simulink model "gm_ZynqBF_2tx_fpga"  (R2018b)
settings: Solver=FixedStepDiscrete  StartTime=0.0  StopTime=10.0  FixedStep=(1/420e3)/128  RelTol=1e-3
undefined symbols (not defined in the file or in its folder): a, b, c
libraries: hdlsllib x873, simulink x349
(part 21 of 40)

== system gm_ZynqBF_2tx_fpga/channel_estimator/peakdetect_ch1/correlator1/rx_ram_q_instance60 ==
  i : Inport  OutDataTypeStr=fixdt(0, 6, 0)  PortDimensions=1  SampleTime=1.86011904761905e-08
  wdata : Inport  Port=2  OutDataTypeStr=fixdt(1, 16, 15)  PortDimensions=1  SampleTime=1.86011904761905e-08
  waddr : Inport  Port=3  OutDataTypeStr=fixdt(0, 9, 0)  PortDimensions=1  SampleTime=1.86011904761905e-08
  we : Inport  Port=4  OutDataTypeStr=fixdt(0, 64, 0)  PortDimensions=1  SampleTime=1.86011904761905e-08
  raddr : Inport  Port=5  OutDataTypeStr=fixdt(0, 10, 0)  PortDimensions=1  SampleTime=1.86011904761905e-08
  shift : Inport  Port=6  OutDataTypeStr=fixdt(0, 6, 0)  PortDimensions=1  SampleTime=1.86011904761905e-08
  Constant : Constant  OutDataTypeStr=fixdt(0, 1, 0)  SampleTime=-1
  Constant1 : Constant  OutDataTypeStr=fixdt(0, 1, 0)  SampleTime=-1
  Relational Operator : RelationalOperator  Operator=<  OutDataTypeStr=boolean  SampleTime=1.86011904761905e-08  RndMeth=Nearest
  Simple Dual Port RAM : hdlsllib/HDL RAMs/Simple Dual Port RAM  ram_size=9
      settings: SourceProductName=HDL Coder  SourceProductBaseCode=HD
  Sum : Sum  AccumDataTypeStr=fixdt(0, 11, 0)  OutDataTypeStr=fixdt(0, 9, 0)  SampleTime=1.86011904761905e-08
  Sum1 : Sum  AccumDataTypeStr=fixdt(0, 7, 0)  OutDataTypeStr=fixdt(0, 9, 0)  SampleTime=1.86011904761905e-08
  Switch : Switch  Criteria=u2 ~= 0  Threshold=double(0)  OutDataTypeStr=fixdt(0, 9, 0)  SampleTime=1.86011904761905e-08
  get_bit : Subsystem
  dout : Outport
  probe : Outport  Port=2
  wires:
  shift/1 -> Relational Operator/2
  raddr/1 -> Switch/3, Sum/2
  we/1 -> get_bit/1(u)
  waddr/1 -> Simple Dual Port RAM/2
  wdata/1 -> Simple Dual Port RAM/1
  i/1 -> Sum1/1, Relational Operator/1
  Constant/1 -> Sum/1
  Constant1/1 -> Sum1/2
  Relational Operator/1 -> Switch/2
  Simple Dual Port RAM/1 -> dout/1
  Sum/1 -> Switch/1
  Sum1/1 -> get_bit/2(ind)
  Switch/1 -> Simple Dual Port RAM/4, probe/1
  get_bit/1(y) -> Simple Dual Port RAM/3

== system gm_ZynqBF_2tx_fpga/channel_estimator/peakdetect_ch1/correlator1/rx_ram_q_instance61 ==
  i : Inport  OutDataTypeStr=fixdt(0, 6, 0)  PortDimensions=1  SampleTime=1.86011904761905e-08
  wdata : Inport  Port=2  OutDataTypeStr=fixdt(1, 16, 15)  PortDimensions=1  SampleTime=1.86011904761905e-08
  waddr : Inport  Port=3  OutDataTypeStr=fixdt(0, 9, 0)  PortDimensions=1  SampleTime=1.86011904761905e-08
  we : Inport  Port=4  OutDataTypeStr=fixdt(0, 64, 0)  PortDimensions=1  SampleTime=1.86011904761905e-08
  raddr : Inport  Port=5  OutDataTypeStr=fixdt(0, 10, 0)  PortDimensions=1  SampleTime=1.86011904761905e-08
  shift : Inport  Port=6  OutDataTypeStr=fixdt(0, 6, 0)  PortDimensions=1  SampleTime=1.86011904761905e-08
  Constant : Constant  OutDataTypeStr=fixdt(0, 1, 0)  SampleTime=-1
  Constant1 : Constant  OutDataTypeStr=fixdt(0, 1, 0)  SampleTime=-1
  Relational Operator : RelationalOperator  Operator=<  OutDataTypeStr=boolean  SampleTime=1.86011904761905e-08  RndMeth=Nearest
  Simple Dual Port RAM : hdlsllib/HDL RAMs/Simple Dual Port RAM  ram_size=9
      settings: SourceProductName=HDL Coder  SourceProductBaseCode=HD
  Sum : Sum  AccumDataTypeStr=fixdt(0, 11, 0)  OutDataTypeStr=fixdt(0, 9, 0)  SampleTime=1.86011904761905e-08
  Sum1 : Sum  AccumDataTypeStr=fixdt(0, 7, 0)  OutDataTypeStr=fixdt(0, 9, 0)  SampleTime=1.86011904761905e-08
  Switch : Switch  Criteria=u2 ~= 0  Threshold=double(0)  OutDataTypeStr=fixdt(0, 9, 0)  SampleTime=1.86011904761905e-08
  get_bit : Subsystem
  dout : Outport
  probe : Outport  Port=2
  wires:
  shift/1 -> Relational Operator/2
  raddr/1 -> Switch/3, Sum/2
  we/1 -> get_bit/1(u)
  waddr/1 -> Simple Dual Port RAM/2
  wdata/1 -> Simple Dual Port RAM/1
  i/1 -> Sum1/1, Relational Operator/1
  Constant/1 -> Sum/1
  Constant1/1 -> Sum1/2
  Relational Operator/1 -> Switch/2
  Simple Dual Port RAM/1 -> dout/1
  Sum/1 -> Switch/1
  Sum1/1 -> get_bit/2(ind)
  Switch/1 -> Simple Dual Port RAM/4, probe/1
  get_bit/1(y) -> Simple Dual Port RAM/3

== system gm_ZynqBF_2tx_fpga/channel_estimator/peakdetect_ch1/correlator1/rx_ram_q_instance62 ==
  i : Inport  OutDataTypeStr=fixdt(0, 6, 0)  PortDimensions=1  SampleTime=1.86011904761905e-08
  wdata : Inport  Port=2  OutDataTypeStr=fixdt(1, 16, 15)  PortDimensions=1  SampleTime=1.86011904761905e-08
  waddr : Inport  Port=3  OutDataTypeStr=fixdt(0, 9, 0)  PortDimensions=1  SampleTime=1.86011904761905e-08
  we : Inport  Port=4  OutDataTypeStr=fixdt(0, 64, 0)  PortDimensions=1  SampleTime=1.86011904761905e-08
  raddr : Inport  Port=5  OutDataTypeStr=fixdt(0, 10, 0)  PortDimensions=1  SampleTime=1.86011904761905e-08
  shift : Inport  Port=6  OutDataTypeStr=fixdt(0, 6, 0)  PortDimensions=1  SampleTime=1.86011904761905e-08
  Constant : Constant  OutDataTypeStr=fixdt(0, 1, 0)  SampleTime=-1
  Constant1 : Constant  OutDataTypeStr=fixdt(0, 1, 0)  SampleTime=-1
  Relational Operator : RelationalOperator  Operator=<  OutDataTypeStr=boolean  SampleTime=1.86011904761905e-08  RndMeth=Nearest
  Simple Dual Port RAM : hdlsllib/HDL RAMs/Simple Dual Port RAM  ram_size=9
      settings: SourceProductName=HDL Coder  SourceProductBaseCode=HD
  Sum : Sum  AccumDataTypeStr=fixdt(0, 11, 0)  OutDataTypeStr=fixdt(0, 9, 0)  SampleTime=1.86011904761905e-08
  Sum1 : Sum  AccumDataTypeStr=fixdt(0, 7, 0)  OutDataTypeStr=fixdt(0, 9, 0)  SampleTime=1.86011904761905e-08
  Switch : Switch  Criteria=u2 ~= 0  Threshold=double(0)  OutDataTypeStr=fixdt(0, 9, 0)  SampleTime=1.86011904761905e-08
  get_bit : Subsystem
  dout : Outport
  probe : Outport  Port=2
  wires:
  shift/1 -> Relational Operator/2
  raddr/1 -> Switch/3, Sum/2
  we/1 -> get_bit/1(u)
  waddr/1 -> Simple Dual Port RAM/2
  wdata/1 -> Simple Dual Port RAM/1
  i/1 -> Sum1/1, Relational Operator/1
  Constant/1 -> Sum/1
  Constant1/1 -> Sum1/2
  Relational Operator/1 -> Switch/2
  Simple Dual Port RAM/1 -> dout/1
  Sum/1 -> Switch/1
  Sum1/1 -> get_bit/2(ind)
  Switch/1 -> Simple Dual Port RAM/4, probe/1
  get_bit/1(y) -> Simple Dual Port RAM/3

== system gm_ZynqBF_2tx_fpga/channel_estimator/peakdetect_ch1/correlator1/rx_ram_q_instance63 ==
  i : Inport  OutDataTypeStr=fixdt(0, 6, 0)  PortDimensions=1  SampleTime=1.86011904761905e-08
  wdata : Inport  Port=2  OutDataTypeStr=fixdt(1, 16, 15)  PortDimensions=1  SampleTime=1.86011904761905e-08
  waddr : Inport  Port=3  OutDataTypeStr=fixdt(0, 9, 0)  PortDimensions=1  SampleTime=1.86011904761905e-08
  we : Inport  Port=4  OutDataTypeStr=fixdt(0, 64, 0)  PortDimensions=1  SampleTime=1.86011904761905e-08
  raddr : Inport  Port=5  OutDataTypeStr=fixdt(0, 10, 0)  PortDimensions=1  SampleTime=1.86011904761905e-08
  shift : Inport  Port=6  OutDataTypeStr=fixdt(0, 6, 0)  PortDimensions=1  SampleTime=1.86011904761905e-08
  Constant : Constant  OutDataTypeStr=fixdt(0, 1, 0)  SampleTime=-1
  Constant1 : Constant  OutDataTypeStr=fixdt(0, 1, 0)  SampleTime=-1
  Relational Operator : RelationalOperator  Operator=<  OutDataTypeStr=boolean  SampleTime=1.86011904761905e-08  RndMeth=Nearest
  Simple Dual Port RAM : hdlsllib/HDL RAMs/Simple Dual Port RAM  ram_size=9
      settings: SourceProductName=HDL Coder  SourceProductBaseCode=HD
  Sum : Sum  AccumDataTypeStr=fixdt(0, 11, 0)  OutDataTypeStr=fixdt(0, 9, 0)  SampleTime=1.86011904761905e-08
  Sum1 : Sum  AccumDataTypeStr=fixdt(0, 7, 0)  OutDataTypeStr=fixdt(0, 9, 0)  SampleTime=1.86011904761905e-08
  Switch : Switch  Criteria=u2 ~= 0  Threshold=double(0)  OutDataTypeStr=fixdt(0, 9, 0)  SampleTime=1.86011904761905e-08
  get_bit : Subsystem
  dout : Outport
  probe : Outport  Port=2
  wires:
  shift/1 -> Relational Operator/2
  raddr/1 -> Switch/3, Sum/2
  we/1 -> get_bit/1(u)
  waddr/1 -> Simple Dual Port RAM/2
  wdata/1 -> Simple Dual Port RAM/1
  i/1 -> Sum1/1, Relational Operator/1
  Constant/1 -> Sum/1
  Constant1/1 -> Sum1/2
  Relational Operator/1 -> Switch/2
  Simple Dual Port RAM/1 -> dout/1
  Sum/1 -> Switch/1
  Sum1/1 -> get_bit/2(ind)
  Switch/1 -> Simple Dual Port RAM/4, probe/1
  get_bit/1(y) -> Simple Dual Port RAM/3

== system gm_ZynqBF_2tx_fpga/channel_estimator/peakdetect_ch1/correlator1/rx_ram_q_instance64 ==
  i : Inport  OutDataTypeStr=fixdt(0, 6, 0)  PortDimensions=1  SampleTime=1.86011904761905e-08
  wdata : Inport  Port=2  OutDataTypeStr=fixdt(1, 16, 15)  PortDimensions=1  SampleTime=1.86011904761905e-08
  waddr : Inport  Port=3  OutDataTypeStr=fixdt(0, 9, 0)  PortDimensions=1  SampleTime=1.86011904761905e-08
  we : Inport  Port=4  OutDataTypeStr=fixdt(0, 64, 0)  PortDimensions=1  SampleTime=1.86011904761905e-08
  raddr : Inport  Port=5  OutDataTypeStr=fixdt(0, 10, 0)  PortDimensions=1  SampleTime=1.86011904761905e-08
  shift : Inport  Port=6  OutDataTypeStr=fixdt(0, 6, 0)  PortDimensions=1  SampleTime=1.86011904761905e-08
  Constant : Constant  OutDataTypeStr=fixdt(0, 1, 0)  SampleTime=-1
  Constant1 : Constant  OutDataTypeStr=fixdt(0, 1, 0)  SampleTime=-1
  Relational Operator : RelationalOperator  Operator=<  OutDataTypeStr=boolean  SampleTime=1.86011904761905e-08  RndMeth=Nearest
  Simple Dual Port RAM : hdlsllib/HDL RAMs/Simple Dual Port RAM  ram_size=9
      settings: SourceProductName=HDL Coder  SourceProductBaseCode=HD
  Sum : Sum  AccumDataTypeStr=fixdt(0, 11, 0)  OutDataTypeStr=fixdt(0, 9, 0)  SampleTime=1.86011904761905e-08
  Sum1 : Sum  AccumDataTypeStr=fixdt(0, 7, 0)  OutDataTypeStr=fixdt(0, 9, 0)  SampleTime=1.86011904761905e-08
  Switch : Switch  Criteria=u2 ~= 0  Threshold=double(0)  OutDataTypeStr=fixdt(0, 9, 0)  SampleTime=1.86011904761905e-08
  get_bit : Subsystem
  dout : Outport
  probe : Outport  Port=2
  wires:
  shift/1 -> Relational Operator/2
  raddr/1 -> Switch/3, Sum/2
  we/1 -> get_bit/1(u)
  waddr/1 -> Simple Dual Port RAM/2
  wdata/1 -> Simple Dual Port RAM/1
  i/1 -> Sum1/1, Relational Operator/1
  Constant/1 -> Sum/1
  Constant1/1 -> Sum1/2
  Relational Operator/1 -> Switch/2
  Simple Dual Port RAM/1 -> dout/1
  Sum/1 -> Switch/1
  Sum1/1 -> get_bit/2(ind)
  Switch/1 -> Simple Dual Port RAM/4, probe/1
  get_bit/1(y) -> Simple Dual Port RAM/3

== system gm_ZynqBF_2tx_fpga/channel_estimator/peakdetect_ch1/correlator1/rx_ram_q_instance7 ==
  i : Inport  OutDataTypeStr=fixdt(0, 6, 0)  PortDimensions=1  SampleTime=1.86011904761905e-08
  wdata : Inport  Port=2  OutDataTypeStr=fixdt(1, 16, 15)  PortDimensions=1  SampleTime=1.86011904761905e-08
  waddr : Inport  Port=3  OutDataTypeStr=fixdt(0, 9, 0)  PortDimensions=1  SampleTime=1.86011904761905e-08
  we : Inport  Port=4  OutDataTypeStr=fixdt(0, 64, 0)  PortDimensions=1  SampleTime=1.86011904761905e-08
  raddr : Inport  Port=5  OutDataTypeStr=fixdt(0, 10, 0)  PortDimensions=1  SampleTime=1.86011904761905e-08
  shift : Inport  Port=6  OutDataTypeStr=fixdt(0, 6, 0)  PortDimensions=1  SampleTime=1.86011904761905e-08
  Constant : Constant  OutDataTypeStr=fixdt(0, 1, 0)  SampleTime=-1
  Constant1 : Constant  OutDataTypeStr=fixdt(0, 1, 0)  SampleTime=-1
  Relational Operator : RelationalOperator  Operator=<  OutDataTypeStr=boolean  SampleTime=1.86011904761905e-08  RndMeth=Nearest
  Simple Dual Port RAM : hdlsllib/HDL RAMs/Simple Dual Port RAM  ram_size=9
      settings: SourceProductName=HDL Coder  SourceProductBaseCode=HD
  Sum : Sum  AccumDataTypeStr=fixdt(0, 11, 0)  OutDataTypeStr=fixdt(0, 9, 0)  SampleTime=1.86011904761905e-08
  Sum1 : Sum  AccumDataTypeStr=fixdt(0, 7, 0)  OutDataTypeStr=fixdt(0, 9, 0)  SampleTime=1.86011904761905e-08
  Switch : Switch  Criteria=u2 ~= 0  Threshold=double(0)  OutDataTypeStr=fixdt(0, 9, 0)  SampleTime=1.86011904761905e-08
  get_bit : Subsystem
  dout : Outport
  probe : Outport  Port=2
  wires:
  shift/1 -> Relational Operator/2
  raddr/1 -> Switch/3, Sum/2
  we/1 -> get_bit/1(u)
  waddr/1 -> Simple Dual Port RAM/2
  wdata/1 -> Simple Dual Port RAM/1
  i/1 -> Sum1/1, Relational Operator/1
  Constant/1 -> Sum/1
  Constant1/1 -> Sum1/2
  Relational Operator/1 -> Switch/2
  Simple Dual Port RAM/1 -> dout/1
  Sum/1 -> Switch/1
  Sum1/1 -> get_bit/2(ind)
  Switch/1 -> Simple Dual Port RAM/4, probe/1
  get_bit/1(y) -> Simple Dual Port RAM/3

== system gm_ZynqBF_2tx_fpga/channel_estimator/peakdetect_ch1/correlator1/rx_ram_q_instance8 ==
  i : Inport  OutDataTypeStr=fixdt(0, 6, 0)  PortDimensions=1  SampleTime=1.86011904761905e-08
  wdata : Inport  Port=2  OutDataTypeStr=fixdt(1, 16, 15)  PortDimensions=1  SampleTime=1.86011904761905e-08
  waddr : Inport  Port=3  OutDataTypeStr=fixdt(0, 9, 0)  PortDimensions=1  SampleTime=1.86011904761905e-08
  we : Inport  Port=4  OutDataTypeStr=fixdt(0, 64, 0)  PortDimensions=1  SampleTime=1.86011904761905e-08
  raddr : Inport  Port=5  OutDataTypeStr=fixdt(0, 10, 0)  PortDimensions=1  SampleTime=1.86011904761905e-08
  shift : Inport  Port=6  OutDataTypeStr=fixdt(0, 6, 0)  PortDimensions=1  SampleTime=1.86011904761905e-08
  Constant : Constant  OutDataTypeStr=fixdt(0, 1, 0)  SampleTime=-1
  Constant1 : Constant  OutDataTypeStr=fixdt(0, 1, 0)  SampleTime=-1
  Relational Operator : RelationalOperator  Operator=<  OutDataTypeStr=boolean  SampleTime=1.86011904761905e-08  RndMeth=Nearest
  Simple Dual Port RAM : hdlsllib/HDL RAMs/Simple Dual Port RAM  ram_size=9
      settings: SourceProductName=HDL Coder  SourceProductBaseCode=HD
  Sum : Sum  AccumDataTypeStr=fixdt(0, 11, 0)  OutDataTypeStr=fixdt(0, 9, 0)  SampleTime=1.86011904761905e-08
  Sum1 : Sum  AccumDataTypeStr=fixdt(0, 7, 0)  OutDataTypeStr=fixdt(0, 9, 0)  SampleTime=1.86011904761905e-08
  Switch : Switch  Criteria=u2 ~= 0  Threshold=double(0)  OutDataTypeStr=fixdt(0, 9, 0)  SampleTime=1.86011904761905e-08
  get_bit : Subsystem
  dout : Outport
  probe : Outport  Port=2
  wires:
  shift/1 -> Relational Operator/2
  raddr/1 -> Switch/3, Sum/2
  we/1 -> get_bit/1(u)
  waddr/1 -> Simple Dual Port RAM/2
  wdata/1 -> Simple Dual Port RAM/1
  i/1 -> Sum1/1, Relational Operator/1
  Constant/1 -> Sum/1
  Constant1/1 -> Sum1/2
  Relational Operator/1 -> Switch/2
  Simple Dual Port RAM/1 -> dout/1
  Sum/1 -> Switch/1
  Sum1/1 -> get_bit/2(ind)
  Switch/1 -> Simple Dual Port RAM/4, probe/1
  get_bit/1(y) -> Simple Dual Port RAM/3

== system gm_ZynqBF_2tx_fpga/channel_estimator/peakdetect_ch1/correlator1/rx_ram_q_instance9 ==
  i : Inport  OutDataTypeStr=fixdt(0, 6, 0)  PortDimensions=1  SampleTime=1.86011904761905e-08
  wdata : Inport  Port=2  OutDataTypeStr=fixdt(1, 16, 15)  PortDimensions=1  SampleTime=1.86011904761905e-08
  waddr : Inport  Port=3  OutDataTypeStr=fixdt(0, 9, 0)  PortDimensions=1  SampleTime=1.86011904761905e-08
  we : Inport  Port=4  OutDataTypeStr=fixdt(0, 64, 0)  PortDimensions=1  SampleTime=1.86011904761905e-08
  raddr : Inport  Port=5  OutDataTypeStr=fixdt(0, 10, 0)  PortDimensions=1  SampleTime=1.86011904761905e-08
  shift : Inport  Port=6  OutDataTypeStr=fixdt(0, 6, 0)  PortDimensions=1  SampleTime=1.86011904761905e-08
  Constant : Constant  OutDataTypeStr=fixdt(0, 1, 0)  SampleTime=-1
  Constant1 : Constant  OutDataTypeStr=fixdt(0, 1, 0)  SampleTime=-1
  Relational Operator : RelationalOperator  Operator=<  OutDataTypeStr=boolean  SampleTime=1.86011904761905e-08  RndMeth=Nearest
  Simple Dual Port RAM : hdlsllib/HDL RAMs/Simple Dual Port RAM  ram_size=9
      settings: SourceProductName=HDL Coder  SourceProductBaseCode=HD
  Sum : Sum  AccumDataTypeStr=fixdt(0, 11, 0)  OutDataTypeStr=fixdt(0, 9, 0)  SampleTime=1.86011904761905e-08
  Sum1 : Sum  AccumDataTypeStr=fixdt(0, 7, 0)  OutDataTypeStr=fixdt(0, 9, 0)  SampleTime=1.86011904761905e-08
  Switch : Switch  Criteria=u2 ~= 0  Threshold=double(0)  OutDataTypeStr=fixdt(0, 9, 0)  SampleTime=1.86011904761905e-08
  get_bit : Subsystem
  dout : Outport
  probe : Outport  Port=2
  wires:
  shift/1 -> Relational Operator/2
  raddr/1 -> Switch/3, Sum/2
  we/1 -> get_bit/1(u)
  waddr/1 -> Simple Dual Port RAM/2
  wdata/1 -> Simple Dual Port RAM/1
  i/1 -> Sum1/1, Relational Operator/1
  Constant/1 -> Sum/1
  Constant1/1 -> Sum1/2
  Relational Operator/1 -> Switch/2
  Simple Dual Port RAM/1 -> dout/1
  Sum/1 -> Switch/1
  Sum1/1 -> get_bit/2(ind)
  Switch/1 -> Simple Dual Port RAM/4, probe/1
  get_bit/1(y) -> Simple Dual Port RAM/3

== system gm_ZynqBF_2tx_fpga/channel_estimator/peakdetect_ch1/correlator1/shift_rx ==
  u : Inport  OutDataTypeStr=fixdt(1, 16, 15)  PortDimensions=[64]  SampleTime=1.86011904761905e-08
  shift : Inport  Port=2  OutDataTypeStr=fixdt(0, 6, 0)  PortDimensions=1  SampleTime=1.86011904761905e-08
  shift_rx : MATLAB Function  TreatAsAtomicUnit=on
  y : Outport
  wires:
  u/1 -> shift_rx/1(u)
  shift/1 -> shift_rx/2(shift)
  shift_rx/1(y) -> y/1

== system gm_ZynqBF_2tx_fpga/channel_estimator/peakdetect_ch1/correlator1/shift_rx1 ==
  u : Inport  OutDataTypeStr=fixdt(1, 16, 15)  PortDimensions=[64]  SampleTime=1.86011904761905e-08
  shift : Inport  Port=2  OutDataTypeStr=fixdt(0, 6, 0)  PortDimensions=1  SampleTime=1.86011904761905e-08
  shift_rx : MATLAB Function  TreatAsAtomicUnit=on
  y : Outport
  wires:
  shift_rx/1(y) -> y/1
  shift/1 -> shift_rx/2(shift)
  u/1 -> shift_rx/1(u)

== system gm_ZynqBF_2tx_fpga/channel_estimator/peakdetect_ch1/correlator1/sum_elements_i_instance1 ==
  din : Inport  OutDataTypeStr=fixdt(1, 32, 16)  PortDimensions=[8]  SampleTime=1.86011904761905e-08
  start : Inport  Port=2  OutDataTypeStr=boolean  PortDimensions=1  SampleTime=1.86011904761905e-08
  Add : Sum  AccumDataTypeStr=fixdt(1, 33, 16)  OutDataTypeStr=fixdt(1, 32, 16)  SampleTime=1.86011904761905e-08
  Compare To Constant1 : simulink/Logic and Bit Operations/Compare To Constant  relop===  const=fi(0,0,3,0,'hex','7')  OutDataTypeStr=boolean
  Compare To Constant2 : simulink/Logic and Bit Operations/Compare To Constant  relop===  const=fi(0,0,1,0,'hex','1')  OutDataTypeStr=boolean
  Constant : Constant  Value=0  OutDataTypeStr=fixdt(1, 32, 16)  SampleTime=-1
  Constant1 : Constant  Value=0  OutDataTypeStr=fixdt(1, 16, 15)  SampleTime=-1
  Data Type Conversion : DataTypeConversion  OutDataTypeStr=uint8  SampleTime=1.86011904761905e-08
  Delay1 : Delay  DelayLength=double(1)  InitialCondition=0  InputProcessing=Inherited  SampleTime=1.86011904761905e-08
  HDL Counter : hdlsllib/Sources/HDL Counter  CountType=Free running  CountInit=double(0)  CountStep=double(1)  CountMax=25  CountFromType=Initial value  CountFrom=double(0)  CountResetPort=on  CountLoadPort=off  CountEnbPort=on  CountDirPort=off  CountDataType=Unsigned  CountWordLen=3  CountFracLen=0  CountSampTime=1.86011904761905e-08
      settings: SourceProductBaseCode=HD
  HDL Counter1 : hdlsllib/Sources/HDL Counter  CountType=Free running  CountInit=double(0)  CountStep=double(1)  CountMax=25  CountFromType=Initial value  CountFrom=double(0)  CountResetPort=off  CountLoadPort=off  CountEnbPort=on  CountDirPort=off  CountDataType=Unsigned  CountWordLen=1  CountFracLen=0  CountSampTime=1.86011904761905e-08
      settings: SourceProductBaseCode=HD
  Logical Operator : Logic  Operator=OR  AllPortsSameDT=off  OutDataTypeStr=boolean  SampleTime=1.86011904761905e-08
  Selector : Selector  IndexMode=Zero-based  SampleTime=1.86011904761905e-08  IndexOptions=Starting index (port)  Indices=double([1 3])  OutputSizes=double(1)
  Switch : Switch  Criteria=u2 ~= 0  Threshold=double(0)  OutDataTypeStr=fixdt(1, 32, 16)  SampleTime=1.86011904761905e-08
  Switch1 : Switch  Criteria=u2 ~= 0  Threshold=double(0)  OutDataTypeStr=fixdt(1, 32, 16)  SampleTime=1.86011904761905e-08
  dout : Outport
  vout : Outport  Port=2
  wires:
  Switch1/1 -> Add/1
  Selector/1 -> Switch1/1
  HDL Counter/1 -> Data Type Conversion/1, Compare To Constant1/1
  Data Type Conversion/1 -> Selector/2
  Constant1/1 -> Switch1/3
  Constant/1 -> Switch/1
  Compare To Constant2/1 -> Switch1/2, HDL Counter/2
  Compare To Constant1/1 -> vout/1, Logical Operator/2
  Add/1 -> dout/1, Delay1/1
  din/1 -> Selector/1
  start/1 -> Logical Operator/1, HDL Counter/1, Switch/2
  Logical Operator/1 -> HDL Counter1/1
  HDL Counter1/1 -> Compare To Constant2/1
  Delay1/1 -> Switch/3
  Switch/1 -> Add/2

== system gm_ZynqBF_2tx_fpga/channel_estimator/peakdetect_ch1/correlator1/sum_elements_i_instance2 ==
  din : Inport  OutDataTypeStr=fixdt(1, 32, 16)  PortDimensions=[8]  SampleTime=1.86011904761905e-08
  start : Inport  Port=2  OutDataTypeStr=boolean  PortDimensions=1  SampleTime=1.86011904761905e-08
  Add : Sum  AccumDataTypeStr=fixdt(1, 33, 16)  OutDataTypeStr=fixdt(1, 32, 16)  SampleTime=1.86011904761905e-08
  Compare To Constant1 : simulink/Logic and Bit Operations/Compare To Constant  relop===  const=fi(0,0,3,0,'hex','7')  OutDataTypeStr=boolean
  Compare To Constant2 : simulink/Logic and Bit Operations/Compare To Constant  relop===  const=fi(0,0,1,0,'hex','1')  OutDataTypeStr=boolean
  Constant : Constant  Value=0  OutDataTypeStr=fixdt(1, 32, 16)  SampleTime=-1
  Constant1 : Constant  Value=0  OutDataTypeStr=fixdt(1, 16, 15)  SampleTime=-1
  Data Type Conversion : DataTypeConversion  OutDataTypeStr=uint8  SampleTime=1.86011904761905e-08
  Delay1 : Delay  DelayLength=double(1)  InitialCondition=0  InputProcessing=Inherited  SampleTime=1.86011904761905e-08
  HDL Counter : hdlsllib/Sources/HDL Counter  CountType=Free running  CountInit=double(0)  CountStep=double(1)  CountMax=25  CountFromType=Initial value  CountFrom=double(0)  CountResetPort=on  CountLoadPort=off  CountEnbPort=on  CountDirPort=off  CountDataType=Unsigned  CountWordLen=3  CountFracLen=0  CountSampTime=1.86011904761905e-08
      settings: SourceProductBaseCode=HD
  HDL Counter1 : hdlsllib/Sources/HDL Counter  CountType=Free running  CountInit=double(0)  CountStep=double(1)  CountMax=25  CountFromType=Initial value  CountFrom=double(0)  CountResetPort=off  CountLoadPort=off  CountEnbPort=on  CountDirPort=off  CountDataType=Unsigned  CountWordLen=1  CountFracLen=0  CountSampTime=1.86011904761905e-08
      settings: SourceProductBaseCode=HD
  Logical Operator : Logic  Operator=OR  AllPortsSameDT=off  OutDataTypeStr=boolean  SampleTime=1.86011904761905e-08
  Selector : Selector  IndexMode=Zero-based  SampleTime=1.86011904761905e-08  IndexOptions=Starting index (port)  Indices=double([1 3])  OutputSizes=double(1)
  Switch : Switch  Criteria=u2 ~= 0  Threshold=double(0)  OutDataTypeStr=fixdt(1, 32, 16)  SampleTime=1.86011904761905e-08
  Switch1 : Switch  Criteria=u2 ~= 0  Threshold=double(0)  OutDataTypeStr=fixdt(1, 32, 16)  SampleTime=1.86011904761905e-08
  dout : Outport
  vout : Outport  Port=2
  wires:
  Switch/1 -> Add/2
  Delay1/1 -> Switch/3
  HDL Counter1/1 -> Compare To Constant2/1
  Logical Operator/1 -> HDL Counter1/1
  start/1 -> Switch/2, HDL Counter/1, Logical Operator/1
  din/1 -> Selector/1
  Add/1 -> Delay1/1, dout/1
  Compare To Constant1/1 -> Logical Operator/2, vout/1
  Compare To Constant2/1 -> HDL Counter/2, Switch1/2
  Constant/1 -> Switch/1
  Constant1/1 -> Switch1/3
  Data Type Conversion/1 -> Selector/2
  HDL Counter/1 -> Compare To Constant1/1, Data Type Conversion/1
  Selector/1 -> Switch1/1
  Switch1/1 -> Add/1

== system gm_ZynqBF_2tx_fpga/channel_estimator/peakdetect_ch1/correlator1/sum_elements_i_instance3 ==
  din : Inport  OutDataTypeStr=fixdt(1, 32, 16)  PortDimensions=[8]  SampleTime=1.86011904761905e-08
  start : Inport  Port=2  OutDataTypeStr=boolean  PortDimensions=1  SampleTime=1.86011904761905e-08
  Add : Sum  AccumDataTypeStr=fixdt(1, 33, 16)  OutDataTypeStr=fixdt(1, 32, 16)  SampleTime=1.86011904761905e-08
  Compare To Constant1 : simulink/Logic and Bit Operations/Compare To Constant  relop===  const=fi(0,0,3,0,'hex','7')  OutDataTypeStr=boolean
  Compare To Constant2 : simulink/Logic and Bit Operations/Compare To Constant  relop===  const=fi(0,0,1,0,'hex','1')  OutDataTypeStr=boolean
  Constant : Constant  Value=0  OutDataTypeStr=fixdt(1, 32, 16)  SampleTime=-1
  Constant1 : Constant  Value=0  OutDataTypeStr=fixdt(1, 16, 15)  SampleTime=-1
  Data Type Conversion : DataTypeConversion  OutDataTypeStr=uint8  SampleTime=1.86011904761905e-08
  Delay1 : Delay  DelayLength=double(1)  InitialCondition=0  InputProcessing=Inherited  SampleTime=1.86011904761905e-08
  HDL Counter : hdlsllib/Sources/HDL Counter  CountType=Free running  CountInit=double(0)  CountStep=double(1)  CountMax=25  CountFromType=Initial value  CountFrom=double(0)  CountResetPort=on  CountLoadPort=off  CountEnbPort=on  CountDirPort=off  CountDataType=Unsigned  CountWordLen=3  CountFracLen=0  CountSampTime=1.86011904761905e-08
      settings: SourceProductBaseCode=HD
  HDL Counter1 : hdlsllib/Sources/HDL Counter  CountType=Free running  CountInit=double(0)  CountStep=double(1)  CountMax=25  CountFromType=Initial value  CountFrom=double(0)  CountResetPort=off  CountLoadPort=off  CountEnbPort=on  CountDirPort=off  CountDataType=Unsigned  CountWordLen=1  CountFracLen=0  CountSampTime=1.86011904761905e-08
      settings: SourceProductBaseCode=HD
  Logical Operator : Logic  Operator=OR  AllPortsSameDT=off  OutDataTypeStr=boolean  SampleTime=1.86011904761905e-08
  Selector : Selector  IndexMode=Zero-based  SampleTime=1.86011904761905e-08  IndexOptions=Starting index (port)  Indices=double([1 3])  OutputSizes=double(1)
  Switch : Switch  Criteria=u2 ~= 0  Threshold=double(0)  OutDataTypeStr=fixdt(1, 32, 16)  SampleTime=1.86011904761905e-08
  Switch1 : Switch  Criteria=u2 ~= 0  Threshold=double(0)  OutDataTypeStr=fixdt(1, 32, 16)  SampleTime=1.86011904761905e-08
  dout : Outport
  vout : Outport  Port=2
  wires:
  Switch/1 -> Add/2
  Delay1/1 -> Switch/3
  HDL Counter1/1 -> Compare To Constant2/1
  Logical Operator/1 -> HDL Counter1/1
  start/1 -> Switch/2, HDL Counter/1, Logical Operator/1
  din/1 -> Selector/1
  Add/1 -> Delay1/1, dout/1
  Compare To Constant1/1 -> Logical Operator/2, vout/1
  Compare To Constant2/1 -> HDL Counter/2, Switch1/2
  Constant/1 -> Switch/1
  Constant1/1 -> Switch1/3
  Data Type Conversion/1 -> Selector/2
  HDL Counter/1 -> Compare To Constant1/1, Data Type Conversion/1
  Selector/1 -> Switch1/1
  Switch1/1 -> Add/1

== system gm_ZynqBF_2tx_fpga/channel_estimator/peakdetect_ch1/correlator1/sum_elements_i_instance4 ==
  din : Inport  OutDataTypeStr=fixdt(1, 32, 16)  PortDimensions=[8]  SampleTime=1.86011904761905e-08
  start : Inport  Port=2  OutDataTypeStr=boolean  PortDimensions=1  SampleTime=1.86011904761905e-08
  Add : Sum  AccumDataTypeStr=fixdt(1, 33, 16)  OutDataTypeStr=fixdt(1, 32, 16)  SampleTime=1.86011904761905e-08
  Compare To Constant1 : simulink/Logic and Bit Operations/Compare To Constant  relop===  const=fi(0,0,3,0,'hex','7')  OutDataTypeStr=boolean
  Compare To Constant2 : simulink/Logic and Bit Operations/Compare To Constant  relop===  const=fi(0,0,1,0,'hex','1')  OutDataTypeStr=boolean
  Constant : Constant  Value=0  OutDataTypeStr=fixdt(1, 32, 16)  SampleTime=-1
  Constant1 : Constant  Value=0  OutDataTypeStr=fixdt(1, 16, 15)  SampleTime=-1
  Data Type Conversion : DataTypeConversion  OutDataTypeStr=uint8  SampleTime=1.86011904761905e-08
  Delay1 : Delay  DelayLength=double(1)  InitialCondition=0  InputProcessing=Inherited  SampleTime=1.86011904761905e-08
  HDL Counter : hdlsllib/Sources/HDL Counter  CountType=Free running  CountInit=double(0)  CountStep=double(1)  CountMax=25  CountFromType=Initial value  CountFrom=double(0)  CountResetPort=on  CountLoadPort=off  CountEnbPort=on  CountDirPort=off  CountDataType=Unsigned  CountWordLen=3  CountFracLen=0  CountSampTime=1.86011904761905e-08
      settings: SourceProductBaseCode=HD
  HDL Counter1 : hdlsllib/Sources/HDL Counter  CountType=Free running  CountInit=double(0)  CountStep=double(1)  CountMax=25  CountFromType=Initial value  CountFrom=double(0)  CountResetPort=off  CountLoadPort=off  CountEnbPort=on  CountDirPort=off  CountDataType=Unsigned  CountWordLen=1  CountFracLen=0  CountSampTime=1.86011904761905e-08
      settings: SourceProductBaseCode=HD
  Logical Operator : Logic  Operator=OR  AllPortsSameDT=off  OutDataTypeStr=boolean  SampleTime=1.86011904761905e-08
  Selector : Selector  IndexMode=Zero-based  SampleTime=1.86011904761905e-08  IndexOptions=Starting index (port)  Indices=double([1 3])  OutputSizes=double(1)
  Switch : Switch  Criteria=u2 ~= 0  Threshold=double(0)  OutDataTypeStr=fixdt(1, 32, 16)  SampleTime=1.86011904761905e-08
  Switch1 : Switch  Criteria=u2 ~= 0  Threshold=double(0)  OutDataTypeStr=fixdt(1, 32, 16)  SampleTime=1.86011904761905e-08
  dout : Outport
  vout : Outport  Port=2
  wires:
  Switch/1 -> Add/2
  Delay1/1 -> Switch/3
  HDL Counter1/1 -> Compare To Constant2/1
  Logical Operator/1 -> HDL Counter1/1
  start/1 -> Switch/2, HDL Counter/1, Logical Operator/1
  din/1 -> Selector/1
  Add/1 -> Delay1/1, dout/1
  Compare To Constant1/1 -> Logical Operator/2, vout/1
  Compare To Constant2/1 -> HDL Counter/2, Switch1/2
  Constant/1 -> Switch/1
  Constant1/1 -> Switch1/3
  Data Type Conversion/1 -> Selector/2
  HDL Counter/1 -> Compare To Constant1/1, Data Type Conversion/1
  Selector/1 -> Switch1/1
  Switch1/1 -> Add/1

== system gm_ZynqBF_2tx_fpga/channel_estimator/peakdetect_ch1/correlator1/sum_elements_i_instance5 ==
  din : Inport  OutDataTypeStr=fixdt(1, 32, 16)  PortDimensions=[8]  SampleTime=1.86011904761905e-08
  start : Inport  Port=2  OutDataTypeStr=boolean  PortDimensions=1  SampleTime=1.86011904761905e-08
  Add : Sum  AccumDataTypeStr=fixdt(1, 33, 16)  OutDataTypeStr=fixdt(1, 32, 16)  SampleTime=1.86011904761905e-08
  Compare To Constant1 : simulink/Logic and Bit Operations/Compare To Constant  relop===  const=fi(0,0,3,0,'hex','7')  OutDataTypeStr=boolean
  Compare To Constant2 : simulink/Logic and Bit Operations/Compare To Constant  relop===  const=fi(0,0,1,0,'hex','1')  OutDataTypeStr=boolean
  Constant : Constant  Value=0  OutDataTypeStr=fixdt(1, 32, 16)  SampleTime=-1
  Constant1 : Constant  Value=0  OutDataTypeStr=fixdt(1, 16, 15)  SampleTime=-1
  Data Type Conversion : DataTypeConversion  OutDataTypeStr=uint8  SampleTime=1.86011904761905e-08
  Delay1 : Delay  DelayLength=double(1)  InitialCondition=0  InputProcessing=Inherited  SampleTime=1.86011904761905e-08
  HDL Counter : hdlsllib/Sources/HDL Counter  CountType=Free running  CountInit=double(0)  CountStep=double(1)  CountMax=25  CountFromType=Initial value  CountFrom=double(0)  CountResetPort=on  CountLoadPort=off  CountEnbPort=on  CountDirPort=off  CountDataType=Unsigned  CountWordLen=3  CountFracLen=0  CountSampTime=1.86011904761905e-08
      settings: SourceProductBaseCode=HD
  HDL Counter1 : hdlsllib/Sources/HDL Counter  CountType=Free running  CountInit=double(0)  CountStep=double(1)  CountMax=25  CountFromType=Initial value  CountFrom=double(0)  CountResetPort=off  CountLoadPort=off  CountEnbPort=on  CountDirPort=off  CountDataType=Unsigned  CountWordLen=1  CountFracLen=0  CountSampTime=1.86011904761905e-08
      settings: SourceProductBaseCode=HD
  Logical Operator : Logic  Operator=OR  AllPortsSameDT=off  OutDataTypeStr=boolean  SampleTime=1.86011904761905e-08
  Selector : Selector  IndexMode=Zero-based  SampleTime=1.86011904761905e-08  IndexOptions=Starting index (port)  Indices=double([1 3])  OutputSizes=double(1)
  Switch : Switch  Criteria=u2 ~= 0  Threshold=double(0)  OutDataTypeStr=fixdt(1, 32, 16)  SampleTime=1.86011904761905e-08
  Switch1 : Switch  Criteria=u2 ~= 0  Threshold=double(0)  OutDataTypeStr=fixdt(1, 32, 16)  SampleTime=1.86011904761905e-08
  dout : Outport
  vout : Outport  Port=2
  wires:
  Switch/1 -> Add/2
  Delay1/1 -> Switch/3
  HDL Counter1/1 -> Compare To Constant2/1
  Logical Operator/1 -> HDL Counter1/1
  start/1 -> Switch/2, HDL Counter/1, Logical Operator/1
  din/1 -> Selector/1
  Add/1 -> Delay1/1, dout/1
  Compare To Constant1/1 -> Logical Operator/2, vout/1
  Compare To Constant2/1 -> HDL Counter/2, Switch1/2
  Constant/1 -> Switch/1
  Constant1/1 -> Switch1/3
  Data Type Conversion/1 -> Selector/2
  HDL Counter/1 -> Compare To Constant1/1, Data Type Conversion/1
  Selector/1 -> Switch1/1
  Switch1/1 -> Add/1

== system gm_ZynqBF_2tx_fpga/channel_estimator/peakdetect_ch1/correlator1/sum_elements_i_instance6 ==
  din : Inport  OutDataTypeStr=fixdt(1, 32, 16)  PortDimensions=[8]  SampleTime=1.86011904761905e-08
  start : Inport  Port=2  OutDataTypeStr=boolean  PortDimensions=1  SampleTime=1.86011904761905e-08
  Add : Sum  AccumDataTypeStr=fixdt(1, 33, 16)  OutDataTypeStr=fixdt(1, 32, 16)  SampleTime=1.86011904761905e-08
  Compare To Constant1 : simulink/Logic and Bit Operations/Compare To Constant  relop===  const=fi(0,0,3,0,'hex','7')  OutDataTypeStr=boolean
  Compare To Constant2 : simulink/Logic and Bit Operations/Compare To Constant  relop===  const=fi(0,0,1,0,'hex','1')  OutDataTypeStr=boolean
  Constant : Constant  Value=0  OutDataTypeStr=fixdt(1, 32, 16)  SampleTime=-1
  Constant1 : Constant  Value=0  OutDataTypeStr=fixdt(1, 16, 15)  SampleTime=-1
  Data Type Conversion : DataTypeConversion  OutDataTypeStr=uint8  SampleTime=1.86011904761905e-08
  Delay1 : Delay  DelayLength=double(1)  InitialCondition=0  InputProcessing=Inherited  SampleTime=1.86011904761905e-08
  HDL Counter : hdlsllib/Sources/HDL Counter  CountType=Free running  CountInit=double(0)  CountStep=double(1)  CountMax=25  CountFromType=Initial value  CountFrom=double(0)  CountResetPort=on  CountLoadPort=off  CountEnbPort=on  CountDirPort=off  CountDataType=Unsigned  CountWordLen=3  CountFracLen=0  CountSampTime=1.86011904761905e-08
      settings: SourceProductBaseCode=HD
  HDL Counter1 : hdlsllib/Sources/HDL Counter  CountType=Free running  CountInit=double(0)  CountStep=double(1)  CountMax=25  CountFromType=Initial value  CountFrom=double(0)  CountResetPort=off  CountLoadPort=off  CountEnbPort=on  CountDirPort=off  CountDataType=Unsigned  CountWordLen=1  CountFracLen=0  CountSampTime=1.86011904761905e-08
      settings: SourceProductBaseCode=HD
  Logical Operator : Logic  Operator=OR  AllPortsSameDT=off  OutDataTypeStr=boolean  SampleTime=1.86011904761905e-08
  Selector : Selector  IndexMode=Zero-based  SampleTime=1.86011904761905e-08  IndexOptions=Starting index (port)  Indices=double([1 3])  OutputSizes=double(1)
  Switch : Switch  Criteria=u2 ~= 0  Threshold=double(0)  OutDataTypeStr=fixdt(1, 32, 16)  SampleTime=1.86011904761905e-08
  Switch1 : Switch  Criteria=u2 ~= 0  Threshold=double(0)  OutDataTypeStr=fixdt(1, 32, 16)  SampleTime=1.86011904761905e-08
  dout : Outport
  vout : Outport  Port=2
  wires:
  Switch/1 -> Add/2
  Delay1/1 -> Switch/3
  HDL Counter1/1 -> Compare To Constant2/1
  Logical Operator/1 -> HDL Counter1/1
  start/1 -> Switch/2, HDL Counter/1, Logical Operator/1
  din/1 -> Selector/1
  Add/1 -> Delay1/1, dout/1
  Compare To Constant1/1 -> Logical Operator/2, vout/1
  Compare To Constant2/1 -> HDL Counter/2, Switch1/2
  Constant/1 -> Switch/1
  Constant1/1 -> Switch1/3
  Data Type Conversion/1 -> Selector/2
  HDL Counter/1 -> Compare To Constant1/1, Data Type Conversion/1
  Selector/1 -> Switch1/1
  Switch1/1 -> Add/1

== system gm_ZynqBF_2tx_fpga/channel_estimator/peakdetect_ch1/correlator1/sum_elements_i_instance7 ==
  din : Inport  OutDataTypeStr=fixdt(1, 32, 16)  PortDimensions=[8]  SampleTime=1.86011904761905e-08
  start : Inport  Port=2  OutDataTypeStr=boolean  PortDimensions=1  SampleTime=1.86011904761905e-08
  Add : Sum  AccumDataTypeStr=fixdt(1, 33, 16)  OutDataTypeStr=fixdt(1, 32, 16)  SampleTime=1.86011904761905e-08
  Compare To Constant1 : simulink/Logic and Bit Operations/Compare To Constant  relop===  const=fi(0,0,3,0,'hex','7')  OutDataTypeStr=boolean
  Compare To Constant2 : simulink/Logic and Bit Operations/Compare To Constant  relop===  const=fi(0,0,1,0,'hex','1')  OutDataTypeStr=boolean
  Constant : Constant  Value=0  OutDataTypeStr=fixdt(1, 32, 16)  SampleTime=-1
  Constant1 : Constant  Value=0  OutDataTypeStr=fixdt(1, 16, 15)  SampleTime=-1
  Data Type Conversion : DataTypeConversion  OutDataTypeStr=uint8  SampleTime=1.86011904761905e-08
  Delay1 : Delay  DelayLength=double(1)  InitialCondition=0  InputProcessing=Inherited  SampleTime=1.86011904761905e-08
  HDL Counter : hdlsllib/Sources/HDL Counter  CountType=Free running  CountInit=double(0)  CountStep=double(1)  CountMax=25  CountFromType=Initial value  CountFrom=double(0)  CountResetPort=on  CountLoadPort=off  CountEnbPort=on  CountDirPort=off  CountDataType=Unsigned  CountWordLen=3  CountFracLen=0  CountSampTime=1.86011904761905e-08
      settings: SourceProductBaseCode=HD
  HDL Counter1 : hdlsllib/Sources/HDL Counter  CountType=Free running  CountInit=double(0)  CountStep=double(1)  CountMax=25  CountFromType=Initial value  CountFrom=double(0)  CountResetPort=off  CountLoadPort=off  CountEnbPort=on  CountDirPort=off  CountDataType=Unsigned  CountWordLen=1  CountFracLen=0  CountSampTime=1.86011904761905e-08
      settings: SourceProductBaseCode=HD
  Logical Operator : Logic  Operator=OR  AllPortsSameDT=off  OutDataTypeStr=boolean  SampleTime=1.86011904761905e-08
  Selector : Selector  IndexMode=Zero-based  SampleTime=1.86011904761905e-08  IndexOptions=Starting index (port)  Indices=double([1 3])  OutputSizes=double(1)
  Switch : Switch  Criteria=u2 ~= 0  Threshold=double(0)  OutDataTypeStr=fixdt(1, 32, 16)  SampleTime=1.86011904761905e-08
  Switch1 : Switch  Criteria=u2 ~= 0  Threshold=double(0)  OutDataTypeStr=fixdt(1, 32, 16)  SampleTime=1.86011904761905e-08
  dout : Outport
  vout : Outport  Port=2
  wires:
  Switch/1 -> Add/2
  Delay1/1 -> Switch/3
  HDL Counter1/1 -> Compare To Constant2/1
  Logical Operator/1 -> HDL Counter1/1
  start/1 -> Switch/2, HDL Counter/1, Logical Operator/1
  din/1 -> Selector/1
  Add/1 -> Delay1/1, dout/1
  Compare To Constant1/1 -> Logical Operator/2, vout/1
  Compare To Constant2/1 -> HDL Counter/2, Switch1/2
  Constant/1 -> Switch/1
  Constant1/1 -> Switch1/3
  Data Type Conversion/1 -> Selector/2
  HDL Counter/1 -> Compare To Constant1/1, Data Type Conversion/1
  Selector/1 -> Switch1/1
  Switch1/1 -> Add/1

== system gm_ZynqBF_2tx_fpga/channel_estimator/peakdetect_ch1/correlator1/sum_elements_i_instance8 ==
  din : Inport  OutDataTypeStr=fixdt(1, 32, 16)  PortDimensions=[8]  SampleTime=1.86011904761905e-08
  start : Inport  Port=2  OutDataTypeStr=boolean  PortDimensions=1  SampleTime=1.86011904761905e-08
  Add : Sum  AccumDataTypeStr=fixdt(1, 33, 16)  OutDataTypeStr=fixdt(1, 32, 16)  SampleTime=1.86011904761905e-08
  Compare To Constant1 : simulink/Logic and Bit Operations/Compare To Constant  relop===  const=fi(0,0,3,0,'hex','7')  OutDataTypeStr=boolean
  Compare To Constant2 : simulink/Logic and Bit Operations/Compare To Constant  relop===  const=fi(0,0,1,0,'hex','1')  OutDataTypeStr=boolean
  Constant : Constant  Value=0  OutDataTypeStr=fixdt(1, 32, 16)  SampleTime=-1
  Constant1 : Constant  Value=0  OutDataTypeStr=fixdt(1, 16, 15)  SampleTime=-1
  Data Type Conversion : DataTypeConversion  OutDataTypeStr=uint8  SampleTime=1.86011904761905e-08
  Delay1 : Delay  DelayLength=double(1)  InitialCondition=0  InputProcessing=Inherited  SampleTime=1.86011904761905e-08
  HDL Counter : hdlsllib/Sources/HDL Counter  CountType=Free running  CountInit=double(0)  CountStep=double(1)  CountMax=25  CountFromType=Initial value  CountFrom=double(0)  CountResetPort=on  CountLoadPort=off  CountEnbPort=on  CountDirPort=off  CountDataType=Unsigned  CountWordLen=3  CountFracLen=0  CountSampTime=1.86011904761905e-08
      settings: SourceProductBaseCode=HD
  HDL Counter1 : hdlsllib/Sources/HDL Counter  CountType=Free running  CountInit=double(0)  CountStep=double(1)  CountMax=25  CountFromType=Initial value  CountFrom=double(0)  CountResetPort=off  CountLoadPort=off  CountEnbPort=on  CountDirPort=off  CountDataType=Unsigned  CountWordLen=1  CountFracLen=0  CountSampTime=1.86011904761905e-08
      settings: SourceProductBaseCode=HD
  Logical Operator : Logic  Operator=OR  AllPortsSameDT=off  OutDataTypeStr=boolean  SampleTime=1.86011904761905e-08
  Selector : Selector  IndexMode=Zero-based  SampleTime=1.86011904761905e-08  IndexOptions=Starting index (port)  Indices=double([1 3])  OutputSizes=double(1)
  Switch : Switch  Criteria=u2 ~= 0  Threshold=double(0)  OutDataTypeStr=fixdt(1, 32, 16)  SampleTime=1.86011904761905e-08
  Switch1 : Switch  Criteria=u2 ~= 0  Threshold=double(0)  OutDataTypeStr=fixdt(1, 32, 16)  SampleTime=1.86011904761905e-08
  dout : Outport
  vout : Outport  Port=2
  wires:
  Switch/1 -> Add/2
  Delay1/1 -> Switch/3
  HDL Counter1/1 -> Compare To Constant2/1
  Logical Operator/1 -> HDL Counter1/1
  start/1 -> Switch/2, HDL Counter/1, Logical Operator/1
  din/1 -> Selector/1
  Add/1 -> Delay1/1, dout/1
  Compare To Constant1/1 -> Logical Operator/2, vout/1
  Compare To Constant2/1 -> HDL Counter/2, Switch1/2
  Constant/1 -> Switch/1
  Constant1/1 -> Switch1/3
  Data Type Conversion/1 -> Selector/2
  HDL Counter/1 -> Compare To Constant1/1, Data Type Conversion/1
  Selector/1 -> Switch1/1
  Switch1/1 -> Add/1

== system gm_ZynqBF_2tx_fpga/channel_estimator/peakdetect_ch1/correlator1/sum_elements_q_instance1 ==
  din : Inport  OutDataTypeStr=fixdt(1, 32, 16)  PortDimensions=[8]  SampleTime=1.86011904761905e-08
  start : Inport  Port=2  OutDataTypeStr=boolean  PortDimensions=1  SampleTime=1.86011904761905e-08
  Add : Sum  AccumDataTypeStr=fixdt(1, 33, 16)  OutDataTypeStr=fixdt(1, 32, 16)  SampleTime=1.86011904761905e-08
  Compare To Constant1 : simulink/Logic and Bit Operations/Compare To Constant  relop===  const=fi(0,0,3,0,'hex','7')  OutDataTypeStr=boolean
  Compare To Constant2 : simulink/Logic and Bit Operations/Compare To Constant  relop===  const=fi(0,0,1,0,'hex','1')  OutDataTypeStr=boolean
  Constant : Constant  Value=0  OutDataTypeStr=fixdt(1, 32, 16)  SampleTime=-1
  Constant1 : Constant  Value=0  OutDataTypeStr=fixdt(1, 16, 15)  SampleTime=-1
  Data Type Conversion : DataTypeConversion  OutDataTypeStr=uint8  SampleTime=1.86011904761905e-08
  Delay1 : Delay  DelayLength=double(1)  InitialCondition=0  InputProcessing=Inherited  SampleTime=1.86011904761905e-08
  HDL Counter : hdlsllib/Sources/HDL Counter  CountType=Free running  CountInit=double(0)  CountStep=double(1)  CountMax=25  CountFromType=Initial value  CountFrom=double(0)  CountResetPort=on  CountLoadPort=off  CountEnbPort=on  CountDirPort=off  CountDataType=Unsigned  CountWordLen=3  CountFracLen=0  CountSampTime=1.86011904761905e-08
      settings: SourceProductBaseCode=HD
  HDL Counter1 : hdlsllib/Sources/HDL Counter  CountType=Free running  CountInit=double(0)  CountStep=double(1)  CountMax=25  CountFromType=Initial value  CountFrom=double(0)  CountResetPort=off  CountLoadPort=off  CountEnbPort=on  CountDirPort=off  CountDataType=Unsigned  CountWordLen=1  CountFracLen=0  CountSampTime=1.86011904761905e-08
      settings: SourceProductBaseCode=HD
  Logical Operator : Logic  Operator=OR  AllPortsSameDT=off  OutDataTypeStr=boolean  SampleTime=1.86011904761905e-08
  Selector : Selector  IndexMode=Zero-based  SampleTime=1.86011904761905e-08  IndexOptions=Starting index (port)  Indices=double([1 3])  OutputSizes=double(1)
  Switch : Switch  Criteria=u2 ~= 0  Threshold=double(0)  OutDataTypeStr=fixdt(1, 32, 16)  SampleTime=1.86011904761905e-08
  Switch1 : Switch  Criteria=u2 ~= 0  Threshold=double(0)  OutDataTypeStr=fixdt(1, 32, 16)  SampleTime=1.86011904761905e-08
  dout : Outport
  vout : Outport  Port=2
  wires:
  Switch/1 -> Add/2
  Delay1/1 -> Switch/3
  HDL Counter1/1 -> Compare To Constant2/1
  Logical Operator/1 -> HDL Counter1/1
  start/1 -> Switch/2, HDL Counter/1, Logical Operator/1
  din/1 -> Selector/1
  Add/1 -> Delay1/1, dout/1
  Compare To Constant1/1 -> Logical Operator/2, vout/1
  Compare To Constant2/1 -> HDL Counter/2, Switch1/2
  Constant/1 -> Switch/1
  Constant1/1 -> Switch1/3
  Data Type Conversion/1 -> Selector/2
  HDL Counter/1 -> Compare To Constant1/1, Data Type Conversion/1
  Selector/1 -> Switch1/1
  Switch1/1 -> Add/1

== system gm_ZynqBF_2tx_fpga/channel_estimator/peakdetect_ch1/correlator1/sum_elements_q_instance2 ==
  din : Inport  OutDataTypeStr=fixdt(1, 32, 16)  PortDimensions=[8]  SampleTime=1.86011904761905e-08
  start : Inport  Port=2  OutDataTypeStr=boolean  PortDimensions=1  SampleTime=1.86011904761905e-08
  Add : Sum  AccumDataTypeStr=fixdt(1, 33, 16)  OutDataTypeStr=fixdt(1, 32, 16)  SampleTime=1.86011904761905e-08
  Compare To Constant1 : simulink/Logic and Bit Operations/Compare To Constant  relop===  const=fi(0,0,3,0,'hex','7')  OutDataTypeStr=boolean
  Compare To Constant2 : simulink/Logic and Bit Operations/Compare To Constant  relop===  const=fi(0,0,1,0,'hex','1')  OutDataTypeStr=boolean
  Constant : Constant  Value=0  OutDataTypeStr=fixdt(1, 32, 16)  SampleTime=-1
  Constant1 : Constant  Value=0  OutDataTypeStr=fixdt(1, 16, 15)  SampleTime=-1
  Data Type Conversion : DataTypeConversion  OutDataTypeStr=uint8  SampleTime=1.86011904761905e-08
  Delay1 : Delay  DelayLength=double(1)  InitialCondition=0  InputProcessing=Inherited  SampleTime=1.86011904761905e-08
  HDL Counter : hdlsllib/Sources/HDL Counter  CountType=Free running  CountInit=double(0)  CountStep=double(1)  CountMax=25  CountFromType=Initial value  CountFrom=double(0)  CountResetPort=on  CountLoadPort=off  CountEnbPort=on  CountDirPort=off  CountDataType=Unsigned  CountWordLen=3  CountFracLen=0  CountSampTime=1.86011904761905e-08
      settings: SourceProductBaseCode=HD
  HDL Counter1 : hdlsllib/Sources/HDL Counter  CountType=Free running  CountInit=double(0)  CountStep=double(1)  CountMax=25  CountFromType=Initial value  CountFrom=double(0)  CountResetPort=off  CountLoadPort=off  CountEnbPort=on  CountDirPort=off  CountDataType=Unsigned  CountWordLen=1  CountFracLen=0  CountSampTime=1.86011904761905e-08
      settings: SourceProductBaseCode=HD
  Logical Operator : Logic  Operator=OR  AllPortsSameDT=off  OutDataTypeStr=boolean  SampleTime=1.86011904761905e-08
  Selector : Selector  IndexMode=Zero-based  SampleTime=1.86011904761905e-08  IndexOptions=Starting index (port)  Indices=double([1 3])  OutputSizes=double(1)
  Switch : Switch  Criteria=u2 ~= 0  Threshold=double(0)  OutDataTypeStr=fixdt(1, 32, 16)  SampleTime=1.86011904761905e-08
  Switch1 : Switch  Criteria=u2 ~= 0  Threshold=double(0)  OutDataTypeStr=fixdt(1, 32, 16)  SampleTime=1.86011904761905e-08
  dout : Outport
  vout : Outport  Port=2
  wires:
  Switch/1 -> Add/2
  Delay1/1 -> Switch/3
  HDL Counter1/1 -> Compare To Constant2/1
  Logical Operator/1 -> HDL Counter1/1
  start/1 -> Switch/2, HDL Counter/1, Logical Operator/1
  din/1 -> Selector/1
  Add/1 -> Delay1/1, dout/1
  Compare To Constant1/1 -> Logical Operator/2, vout/1
  Compare To Constant2/1 -> HDL Counter/2, Switch1/2
  Constant/1 -> Switch/1
  Constant1/1 -> Switch1/3
  Data Type Conversion/1 -> Selector/2
  HDL Counter/1 -> Compare To Constant1/1, Data Type Conversion/1
  Selector/1 -> Switch1/1
  Switch1/1 -> Add/1

== system gm_ZynqBF_2tx_fpga/channel_estimator/peakdetect_ch1/correlator1/sum_elements_q_instance3 ==
  din : Inport  OutDataTypeStr=fixdt(1, 32, 16)  PortDimensions=[8]  SampleTime=1.86011904761905e-08
  start : Inport  Port=2  OutDataTypeStr=boolean  PortDimensions=1  SampleTime=1.86011904761905e-08
  Add : Sum  AccumDataTypeStr=fixdt(1, 33, 16)  OutDataTypeStr=fixdt(1, 32, 16)  SampleTime=1.86011904761905e-08
  Compare To Constant1 : simulink/Logic and Bit Operations/Compare To Constant  relop===  const=fi(0,0,3,0,'hex','7')  OutDataTypeStr=boolean
  Compare To Constant2 : simulink/Logic and Bit Operations/Compare To Constant  relop===  const=fi(0,0,1,0,'hex','1')  OutDataTypeStr=boolean
  Constant : Constant  Value=0  OutDataTypeStr=fixdt(1, 32, 16)  SampleTime=-1
  Constant1 : Constant  Value=0  OutDataTypeStr=fixdt(1, 16, 15)  SampleTime=-1
  Data Type Conversion : DataTypeConversion  OutDataTypeStr=uint8  SampleTime=1.86011904761905e-08
  Delay1 : Delay  DelayLength=double(1)  InitialCondition=0  InputProcessing=Inherited  SampleTime=1.86011904761905e-08
  HDL Counter : hdlsllib/Sources/HDL Counter  CountType=Free running  CountInit=double(0)  CountStep=double(1)  CountMax=25  CountFromType=Initial value  CountFrom=double(0)  CountResetPort=on  CountLoadPort=off  CountEnbPort=on  CountDirPort=off  CountDataType=Unsigned  CountWordLen=3  CountFracLen=0  CountSampTime=1.86011904761905e-08
      settings: SourceProductBaseCode=HD
  HDL Counter1 : hdlsllib/Sources/HDL Counter  CountType=Free running  CountInit=double(0)  CountStep=double(1)  CountMax=25  CountFromType=Initial value  CountFrom=double(0)  CountResetPort=off  CountLoadPort=off  CountEnbPort=on  CountDirPort=off  CountDataType=Unsigned  CountWordLen=1  CountFracLen=0  CountSampTime=1.86011904761905e-08
      settings: SourceProductBaseCode=HD
  Logical Operator : Logic  Operator=OR  AllPortsSameDT=off  OutDataTypeStr=boolean  SampleTime=1.86011904761905e-08
  Selector : Selector  IndexMode=Zero-based  SampleTime=1.86011904761905e-08  IndexOptions=Starting index (port)  Indices=double([1 3])  OutputSizes=double(1)
  Switch : Switch  Criteria=u2 ~= 0  Threshold=double(0)  OutDataTypeStr=fixdt(1, 32, 16)  SampleTime=1.86011904761905e-08
  Switch1 : Switch  Criteria=u2 ~= 0  Threshold=double(0)  OutDataTypeStr=fixdt(1, 32, 16)  SampleTime=1.86011904761905e-08
  dout : Outport
  vout : Outport  Port=2
  wires:
  Switch/1 -> Add/2
  Delay1/1 -> Switch/3
  HDL Counter1/1 -> Compare To Constant2/1
  Logical Operator/1 -> HDL Counter1/1
  start/1 -> Switch/2, HDL Counter/1, Logical Operator/1
  din/1 -> Selector/1
  Add/1 -> Delay1/1, dout/1
  Compare To Constant1/1 -> Logical Operator/2, vout/1
  Compare To Constant2/1 -> HDL Counter/2, Switch1/2
  Constant/1 -> Switch/1
  Constant1/1 -> Switch1/3
  Data Type Conversion/1 -> Selector/2
  HDL Counter/1 -> Compare To Constant1/1, Data Type Conversion/1
  Selector/1 -> Switch1/1
  Switch1/1 -> Add/1
